simulink model "O_CloseLoop_Dynmodel"  (R2016b)
settings: Solver=VariableStepAuto  StartTime=0.0  StopTime=60.0  RelTol=1e-3
values from neighbouring files (symbols this model uses):
  MWS = JT9D_setup_everything_Dyn()    [BP_change_deter_data.m]    (also in JT9D_setup_everything_Dyn.m = input_set_0_0_100(MWS); make_train_data.m; sim_all_loss.m)
undefined symbols (not defined in the file or in its folder): Compressor, Lib_Turbo_Compressor_TMATS, stripchar_TMATS
libraries: Lib_Turbo_Duct_TMATS x5, Lib_Solve_DataOut_TMATS x5, Lib_Solve_OuterLoopIntegrator_TMATS x2, Lib_Turbo_Nozzle_TMATS x2, Lib_Turbo_Shaft_TMATS x2, Lib_Cntrl_FirstOrderActuator_TMATS x1, simulink x1, Lib_Cntrl_SimplePIcontroller_TMATS x1, Lib_Solve_IterNRSolverJC_TMATS x1, Lib_Turbo_Ambient_TMATS x1, Lib_Turbo_Burner_TMATS x1, Lib_Turbo_StaticCalc_TMATS x1
(part 2 of 2)

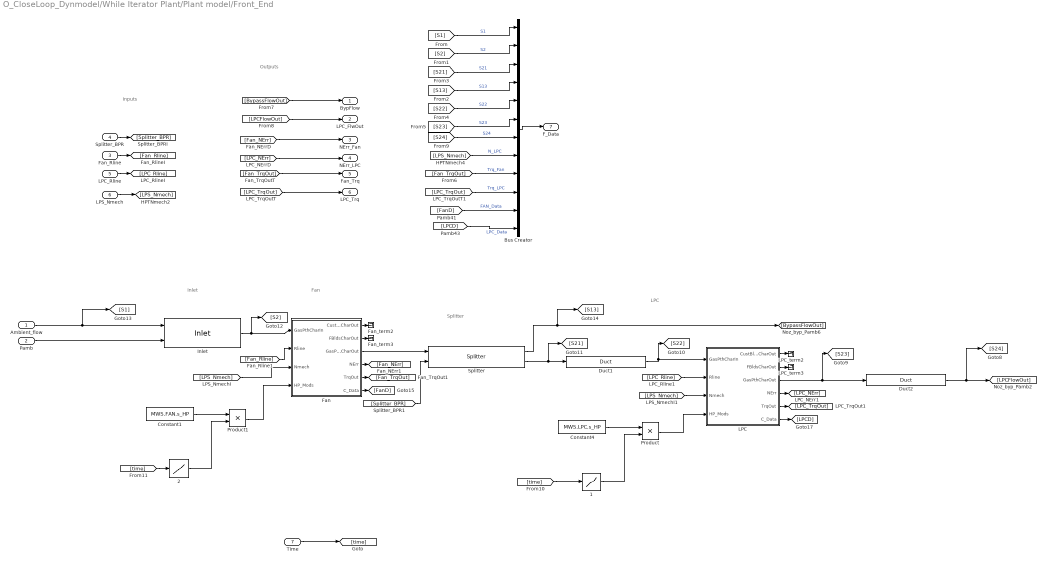
== system O_CloseLoop_Dynmodel/While Iterator Plant/Plant model/Front_End ==
  note: Inlet
  note: Fan
  note: Splitter
  note: LPC
  note: Outputs
  note: Inputs
  Ambient_flow : Inport
  Pamb : Inport  Port=2
  Fan_Rline : Inport  Port=3
  Splitter_BPR : Inport  Port=4
  LPC_Rline : Inport  Port=5
  LPS_Nmech : Inport  Port=6
  Time : Inport  Port=7
  1 : Lookup  InputValues=MWS.HP_in.t  Table=MWS.HP_in.scaled
  2 : Lookup  InputValues=MWS.HP_in.t  Table=MWS.HP_in.scaled
  Bus Creator : BusCreator  Inputs=12
  Constant1 : Constant  Value=MWS.FAN.s_HP
  Constant4 : Constant  Value=MWS.LPC.s_HP
  Duct1 : Lib_Turbo_Duct_TMATS/Duct  dP_M=MWS.Duct.dP1
  Duct2 : Lib_Turbo_Duct_TMATS/Duct  dP_M=MWS.Duct.dP2
  Fan : Subsystem  AncestorBlock=Lib_Turbo_Compressor_TMATS/Compressor  mask(T-MATS: Compressor Library Block){X_C_RlineVec_M=MWS.FAN.RlineVec, Z_C_AlphaVec_M=1, Y_C_Map_NcVec_M=MWS.FAN.NcVec, T_C_Map_WcArray_M=MWS.FAN.WcArray, T_C_Map_PRArray_M=MWS.FAN.PRArray, T_C_Map_EffArray_M=MWS.FAN.EffArray, s_C_Nc_M=MWS.FAN.s_Nc, s_C_Wc_M=MWS.FAN.s_Wc, s_C_PR_M=MWS.FAN.s_PR, s_C_Eff_M=MWS.FAN.s_eff, SL_M=off, Scale_M=none, CBLDEN_M=off, C_CBD_M=0, C_CBFht_M=0.5, C_CBFPt_M=0.5, FBLDEN_M=off, C_FBD_M=0, C_BFht_M=0.5, C_BFPt_M=0.5, DefSMEn_M=on, SRline_M=1, X_C_Map_WcSurgeVec_M=[0 200], T_C_Map_PRSurgeVec_M=[30 30], iDesign_M=MWS.iDes, NcDes_M=1, EffDes_M=0.8675, PRDes_M=1.645, RlineDes_M=2.3706, FVar_M=strcat('iDes_',stripchar_TMATS(gcb),'.bin'), BlkNm_M=double(gcb), HP_M=on}
      mask prompts: X_C_RlineVec_M "X_C_RlineVec_M - Compressor Map Rline Vector (X-axis)(nx1)"; Z_C_AlphaVec_M "Z_C_Map_AlphaVec_M - Compressor Alpha Vector (Z-axis)(rx1)"; Y_C_Map_NcVec_M "Y_C_Map_NcVec_M - Compressor Map Corrected Speed Vector (Y-axis)(mx1)"; T_C_Map_WcArray_M "T_C_Map_WcArray_M - Compressor Map Flow Array (Wc = f(Nc, Rline))(mxn)"; T_C_Map_PRArray_M "T_C_Map_PRArray_M - Compressor Map Pressure Ratio Array (PR = f(Nc, Rline))(mxn)"; T_C_Map_EffArray_M "T_C_Map_EffArray_M - Compressor Map Efficiency Array (Eff = f(Nc, Rline)(mxn)"; s_C_Nc_M "s_C_Nc_M - Corrected Speed Scalar Constant (C_Nc)"; s_C_Wc_M "s_C_Wc_M - Flow Scalar Constant (C_Wc)"; s_C_PR_M "s_C_PR_M - Pressure Ratio Scalar Constant (C_PR)"; s_C_Eff_M "s_C_Eff_M - Efficiency Scalar Constant (C_Eff)"; SL_M "Include surge line"; Scale_M "Scalars"; CBLDEN_M "CBLDEN_M - Customer Bleed Enable [0 - off, 1 - on]"; C_CBD_M "C_CBD_M - Customer or Flow based Bleed Demand[pps] (cbx1)"; C_CBFht_M "C_CBFht_M - Customer or Flow based Bleed Fractional enthalpy[frac] (cbx1)"; C_CBFPt_M "C_CBFPt_M - Customer or Flow based Bleed Fractional Total Pressure[frac] (cbx1)"; FBLDEN_M "FBLDEN_M - Fractional Bleed Enable [0 - off, 1 - on]"; C_FBD_M "C_FBD_M - Fractional Bleed Demand[frac] (bx1)"; C_BFht_M "C_BFht_M - Engine Bleed Fractional Enthalpy[frac] (bx1)"; C_BFPt_M "C_BFPt_M - Engine Bleed Fractional Total Pressure[frac] (bx1)"; DefSMEn_M "DefSMEn_M - Use map default (Rline = 1) surge line"; SRline_M "SRline_M - Rline defined as surge line"; X_C_Map_WcSurgeVec_M "X_C_Map_WcSurgeVec_M - map Compensated flow surge vector (sx1)"; T_C_Map_PRSurgeVec_M "T_C_Map_PRSurgeVec_M - map Surge Line Pressure Ratio vector (sx1)"; iDesign_M "iDesign_M - Design fork (0 - Enable iDes, 1 - Use iDes Scalars, 2 - Use Specified Input Scalars)"; NcDes_M "NcDes_M - map Design Corrected Shaft Speed [rpm]"; EffDes_M "EffDes_M  - Design Efficiency [frac]"; PRDes_M "PRDes_M - Design Pressure Ratio [frac]"; RlineDes_M "RlineDes_M - map Design Rline"; FVar_M "FVar_M - File name for iDes Variables"; BlkNm_M "Block name as double for Simulink output"; HP_M "HP_M - Enable Health Parameter input (3x1 vector)"
      mask help: This block simulates the performance of a compressor using basic thermodynamic equations, properties, and table lookups.
      mask init:
      | MSK_CompInit_TMATS
      mask Help: web(which('Turbo_TMATS_Cmp.html'),'-helpbrowser')
      mask TypeOptions Scale_M: none | user defined | iDesign
      mask Callback CBLDEN_M: MSK_SEC_Enables_TMATS('CBLDEN_M',[14 15 16],'en')
      mask Callback FBLDEN_M: MSK_SEC_Enables_TMATS('FBLDEN_M',[18 19 20],'en')
      mask Callback DefSMEn_M:
      | MSK_SEC_Enables_TMATS('DefSMEn_M',[23 24],'dis')
      | MSK_SEC_Enables_TMATS('DefSMEn_M',[22],'en')
      mask Callback iDesign_M:
      | MSK_SEC_Enables_Ides_TMATS('iDesign_M',[7 8 9 10],'G1')
      | MSK_SEC_Enables_Ides_TMATS('iDesign_M',[26 27 28 29],'G2')
      | MSK_SEC_Enables_Ides_TMATS('iDesign_M',[30],'G3')
      mask DialogControl Control2 Prompt: Plot Map
      mask DialogControl Control2 Callback: MSK_PlotCMap_TMATS()
  Fan_term2 : Terminator
  Fan_term3 : Terminator
  Inlet : Lib_Turbo_Inlet_TMATS/Inlet  eRambase_M=MWS.Inlet.eRamBase  X_eRamVec_M=MWS.Inlet.eRamVec  T_eRamtbl_M=MWS.Inlet.eRamtbl
  LPC : Subsystem  mask(T-MATS: Compressor Library Block){X_C_RlineVec_M=MWS.LPC.RlineVec, Z_C_AlphaVec_M=1, Y_C_Map_NcVec_M=MWS.LPC.NcVec, T_C_Map_WcArray_M=MWS.LPC.WcArray, T_C_Map_PRArray_M=MWS.LPC.PRArray, T_C_Map_EffArray_M=MWS.LPC.EffArray, s_C_Nc_M=MWS.LPC.s_Nc, s_C_Wc_M=MWS.LPC.s_Wc, s_C_PR_M=MWS.LPC.s_PR, s_C_Eff_M=MWS.LPC.s_eff, SL_M=off, Scale_M=none, CBLDEN_M=off, C_CBD_M=0, C_CBFht_M=0.5, C_CBFPt_M=0.5, FBLDEN_M=off, C_FBD_M=0, C_BFht_M=0.5, C_BFPt_M=0.5, DefSMEn_M=on, SRline_M=1, X_C_Map_WcSurgeVec_M=[0 200], T_C_Map_PRSurgeVec_M=[30 30], iDesign_M=MWS.iDes, NcDes_M=0.993, EffDes_M=.8683, PRDes_M=2.488, RlineDes_M=1.7664, FVar_M=strcat('iDes_',stripchar_TMATS(gcb),'.bin'), BlkNm_M=double(gcb), HP_M=on}
      mask prompts: X_C_RlineVec_M "X_C_RlineVec_M - Compressor Map Rline Vector (X-axis)(nx1)"; Z_C_AlphaVec_M "Z_C_Map_AlphaVec_M - Compressor Alpha Vector (Z-axis)(rx1)"; Y_C_Map_NcVec_M "Y_C_Map_NcVec_M - Compressor Map Corrected Speed Vector (Y-axis)(mx1)"; T_C_Map_WcArray_M "T_C_Map_WcArray_M - Compressor Map Flow Array (Wc = f(Nc, Rline))(mxn)"; T_C_Map_PRArray_M "T_C_Map_PRArray_M - Compressor Map Pressure Ratio Array (PR = f(Nc, Rline))(mxn)"; T_C_Map_EffArray_M "T_C_Map_EffArray_M - Compressor Map Efficiency Array (Eff = f(Nc, Rline)(mxn)"; s_C_Nc_M "s_C_Nc_M - Corrected Speed Scalar Constant (C_Nc)"; s_C_Wc_M "s_C_Wc_M - Flow Scalar Constant (C_Wc)"; s_C_PR_M "s_C_PR_M - Pressure Ratio Scalar Constant (C_PR)"; s_C_Eff_M "s_C_Eff_M - Efficiency Scalar Constant (C_Eff)"; SL_M "Include surge line"; Scale_M "Scalars"; CBLDEN_M "CBLDEN_M - Customer Bleed Enable [0 - off, 1 - on]"; C_CBD_M "C_CBD_M - Customer or Flow based Bleed Demand[pps] (cbx1)"; C_CBFht_M "C_CBFht_M - Customer or Flow based Bleed Fractional enthalpy[frac] (cbx1)"; C_CBFPt_M "C_CBFPt_M - Customer or Flow based Bleed Fractional Total Pressure[frac] (cbx1)"; FBLDEN_M "FBLDEN_M - Fractional Bleed Enable [0 - off, 1 - on]"; C_FBD_M "C_FBD_M - Fractional Bleed Demand[frac] (bx1)"; C_BFht_M "C_BFht_M - Engine Bleed Fractional Enthalpy[frac] (bx1)"; C_BFPt_M "C_BFPt_M - Engine Bleed Fractional Total Pressure[frac] (bx1)"; DefSMEn_M "DefSMEn_M - Use map default (Rline = 1) surge line"; SRline_M "SRline_M - Rline defined as surge line"; X_C_Map_WcSurgeVec_M "X_C_Map_WcSurgeVec_M - map Compensated flow surge vector (sx1)"; T_C_Map_PRSurgeVec_M "T_C_Map_PRSurgeVec_M - map Surge Line Pressure Ratio vector (sx1)"; iDesign_M "iDesign_M - Design fork (0 - Enable iDes, 1 - Use iDes Scalars, 2 - Use Specified Input Scalars)"; NcDes_M "NcDes_M - map Design Corrected Shaft Speed [rpm]"; EffDes_M "EffDes_M  - Design Efficiency [frac]"; PRDes_M "PRDes_M - Design Pressure Ratio [frac]"; RlineDes_M "RlineDes_M - map Design Rline"; FVar_M "FVar_M - File name for iDes Variables"; BlkNm_M "Block name as double for Simulink output"; HP_M "HP_M - Enable Health Parameter input (3x1 vector)"
      mask help: This block simulates the performance of a compressor using basic thermodynamic equations, properties, and table lookups.
      mask init:
      | MSK_CompInit_TMATS
      mask Help: web(which('Turbo_TMATS_Cmp.html'),'-helpbrowser')
      mask TypeOptions Scale_M: none | user defined | iDesign
      mask Callback CBLDEN_M: MSK_SEC_Enables_TMATS('CBLDEN_M',[14 15 16],'en')
      mask Callback FBLDEN_M: MSK_SEC_Enables_TMATS('FBLDEN_M',[18 19 20],'en')
      mask Callback DefSMEn_M:
      | MSK_SEC_Enables_TMATS('DefSMEn_M',[23 24],'dis')
      | MSK_SEC_Enables_TMATS('DefSMEn_M',[22],'en')
      mask Callback iDesign_M:
      | MSK_SEC_Enables_Ides_TMATS('iDesign_M',[7 8 9 10],'G1')
      | MSK_SEC_Enables_Ides_TMATS('iDesign_M',[26 27 28 29],'G2')
      | MSK_SEC_Enables_Ides_TMATS('iDesign_M',[30],'G3')
      mask DialogControl Control2 Prompt: Plot Map
      mask DialogControl Control2 Callback: MSK_PlotCMap_TMATS()
  LPC_term2 : Terminator
  LPC_term3 : Terminator
  Product : Product
  Product1 : Product
  Splitter : Lib_Turbo_Splitter_TMATS/Splitter
  BypFlow : Outport
  LPC_FlwOut : Outport  Port=2
  NErr_Fan : Outport  Port=3
  NErr_LPC : Outport  Port=4
  Fan_Trq : Outport  Port=5
  LPC_Trq : Outport  Port=6
  F_Data : Outport  Port=7
  wires:
  [LPCFlowOut] -> LPC_FlwOut/1
  [Splitter_BPR] -> Splitter/2
  Inlet/1 -> [S2], Fan/1(GasPthCharIn)
  [Fan_Rline] -> Fan/2(Rline)
  LPC/2(FBldsCharOut) -> LPC_term3/1
  LPC/4(NErr) -> [LPC_NErr]
  LPC/5(TrqOut) -> [LPC_TrqOut]
  LPC/1(CustBldsCharOut) -> LPC_term2/1
  [LPC_Rline] -> LPC/2(Rline)
  Fan/2(FBldsCharOut) -> Fan_term3/1
  Fan/6(C_Data) -> [FanD]
  Fan/1(CustBldsCharOut) -> Fan_term2/1
  Fan/5(TrqOut) -> [Fan_TrqOut]
  Fan/4(NErr) -> [Fan_NErr]
  Duct1/1 -> LPC/1(GasPthCharIn), [S22]
  Splitter/2 -> [S21], Duct1/1
  Fan/3(GasPthCharOut) -> Splitter/1
  [LPS_Nmech] -> LPC/3(Nmech)
  [LPS_Nmech] -> Fan/3(Nmech)
  [Fan_TrqOut] -> Bus Creator/9  "Trq_Fan"
  LPC/6(C_Data) -> [LPCD]
  Pamb/1 -> Inlet/2
  Ambient_flow/1 -> [S1], Inlet/1
  Fan_Rline/1 -> [Fan_Rline]
  LPS_Nmech/1 -> [LPS_Nmech]
  Splitter_BPR/1 -> [Splitter_BPR]
  LPC_Rline/1 -> [LPC_Rline]
  [S1] -> Bus Creator/1  "S1"
  [FanD] -> Bus Creator/11  "FAN_Data"
  [S22] -> Bus Creator/5  "S22"
  [S23] -> Bus Creator/6  "S23"
  [S21] -> Bus Creator/3  "S21"
  Bus Creator/1 -> F_Data/1
  [LPC_TrqOut] -> Bus Creator/10  "Trq_LPC"
  [LPCD] -> Bus Creator/12  "LPC_Data"
  [S2] -> Bus Creator/2  "S2"
  [LPS_Nmech] -> Bus Creator/8  "N_LPC"
  [S13] -> Bus Creator/4  "S13"
  Splitter/1 -> [S13], [BypassFlowOut]
  LPC/3(GasPthCharOut) -> Duct2/1, [S23]
  [LPC_TrqOut] -> LPC_Trq/1
  [Fan_NErr] -> NErr_Fan/1
  [Fan_TrqOut] -> Fan_Trq/1
  [LPC_NErr] -> NErr_LPC/1
  [BypassFlowOut] -> BypFlow/1
  Duct2/1 -> [LPCFlowOut], [S24]
  [S24] -> Bus Creator/7  "S24"
  Constant4/1 -> Product/1
  Product/1 -> LPC/4(HP_Mods)
  1/1 -> Product/2
  [time] -> 1/1
  Time/1 -> [time]
  Constant1/1 -> Product1/1
  Product1/1 -> Fan/4(HP_Mods)
  2/1 -> Product1/2
  [time] -> 2/1

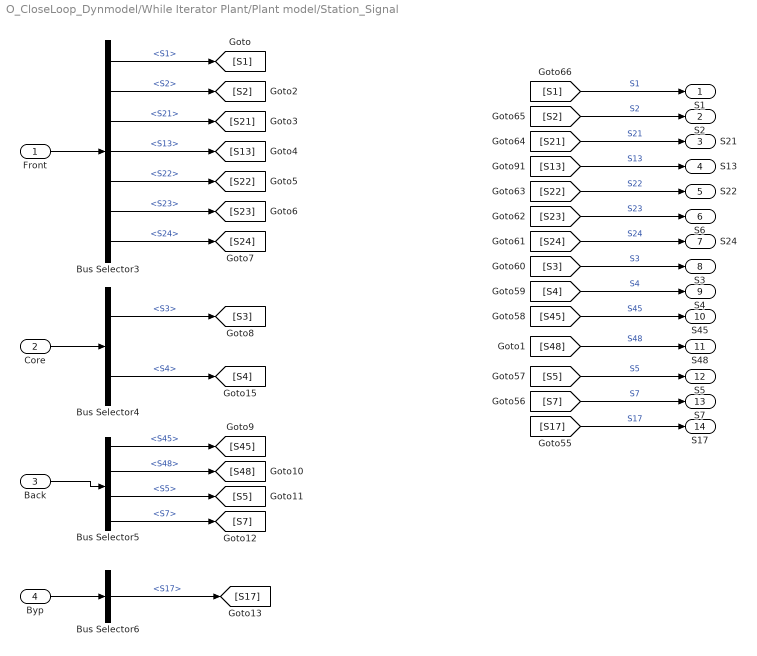
== system O_CloseLoop_Dynmodel/While Iterator Plant/Plant model/Station_Signal ==
  Front : Inport
  Core : Inport  Port=2
  Back : Inport  Port=3
  Byp : Inport  Port=4
  Bus Selector3 : BusSelector  OutputSignals=S1,S2,S21,S13,S22,S23,S24
  Bus Selector4 : BusSelector  OutputSignals=S3,S4
  Bus Selector5 : BusSelector  OutputSignals=S45,S48,S5,S7
  Bus Selector6 : BusSelector  OutputSignals=S17
  S1 : Outport
  S2 : Outport  Port=2
  S21 : Outport  Port=3
  S13 : Outport  Port=4
  S22 : Outport  Port=5
  S6 : Outport  Port=6
  S24 : Outport  Port=7
  S3 : Outport  Port=8
  S4 : Outport  Port=9
  S45 : Outport  Port=10
  S48 : Outport  Port=11
  S5 : Outport  Port=12
  S7 : Outport  Port=13
  S17 : Outport  Port=14
  wires:
  [S21] -> S21/1  "S21"
  [S45] -> S45/1  "S45"
  [S23] -> S6/1  "S23"
  [S7] -> S7/1  "S7"
  [S13] -> S13/1  "S13"
  [S22] -> S22/1  "S22"
  [S3] -> S3/1  "S3"
  [S4] -> S4/1  "S4"
  [S5] -> S5/1  "S5"
  [S17] -> S17/1  "S17"
  [S2] -> S2/1  "S2"
  [S24] -> S24/1  "S24"
  [S1] -> S1/1  "S1"
  Bus Selector4/2 -> [S4]  "<S4>"
  Bus Selector5/4 -> [S7]  "<S7>"
  Core/1 -> Bus Selector4/1
  Bus Selector5/1 -> [S45]  "<S45>"
  Bus Selector6/1 -> [S17]  "<S17>"
  Byp/1 -> Bus Selector6/1
  Bus Selector4/1 -> [S3]  "<S3>"
  Back/1 -> Bus Selector5/1
  Bus Selector5/2 -> [S48]  "<S48>"
  Bus Selector5/3 -> [S5]  "<S5>"
  [S48] -> S48/1  "S48"
  Bus Selector3/4 -> [S13]  "<S13>"
  Bus Selector3/5 -> [S22]  "<S22>"
  Bus Selector3/7 -> [S24]  "<S24>"
  Bus Selector3/3 -> [S21]  "<S21>"
  Bus Selector3/2 -> [S2]  "<S2>"
  Bus Selector3/6 -> [S23]  "<S23>"
  Front/1 -> Bus Selector3/1
  Bus Selector3/1 -> [S1]  "<S1>"

== system O_CloseLoop_Dynmodel/While Iterator Plant/Plant model/Subsystem ==
  BypFlow : Inport
  Pamb : Inport  Port=2
  Bus Creator8 : BusCreator  Inputs=2
  Duct5 : Lib_Turbo_Duct_TMATS/Duct  dP_M=MWS.Duct.dP5
  Noz_byp : Lib_Turbo_Nozzle_TMATS/Nozzle  SWType_M=Convergent  N_TArea_M=MWS.NozB.Ath  N_EArea_M=110.7  N_FL_M=0.00  X_N_TtVec2_M=[300 2000]  T_N_TGArray_M=[1 1]  X_N_PEQPaVec_M=[0 10000]  T_N_CdThArray_M=[1 1]  T_N_CvArray_M=MWS.NozB.CvArray  CfgEn_M=off  T_N_CfgArray_M=[1 1]  X_N_FARVec_M=[0; 0.0050; 0.0100; 0.0150; 0.0200; 0.0250; 0.0300]  T_N_RtArray_M="[0.0686;    0.0686;    0.0686;    0.0686;    0.0686;    0.0686;    0.0686]"  Y_N_TtVec_M=[300 2000]  T_N_MAP_gammaArray_M=[ 1.4 1.4 1.4 1.4 1.4 1.4 1.4; 1.4 1.4 1.4 1.4 1.4 1.4 1.4]  iDesign_M=MWS.iDes  WDes_M=562.61  FVar_M=strcat('iDes_',stripchar_TMATS(gcb),'.bin')
  Noz_byp_term1 : Terminator
  Noz_byp_term3 : Terminator
  NErr_Noz_byp : Outport
  By_Data : Outport  Port=2
  wires:
  Pamb/1 -> Noz_byp/2
  Duct5/1 -> [S17], Noz_byp/1
  Noz_byp/4 -> Noz_byp_term1/1
  Noz_byp/3 -> [Noz_byp_NErr]
  Noz_byp/1 -> Noz_byp_term3/1
  Noz_byp/2 -> [Byp_Fg]
  BypFlow/1 -> Duct5/1
  [S17] -> Bus Creator8/1  "S17"
  Bus Creator8/1 -> By_Data/1
  [Noz_byp_NErr] -> NErr_Noz_byp/1
  [Byp_Fg] -> Bus Creator8/2  "Fg_Byp"

== system O_CloseLoop_Dynmodel/While Iterator Plant/Plant model/Thrust_Calculate ==
  Byp_Fg : Inport
  Core_Fg : Inport  Port=2
  AmbData : Inport  Port=3
  Wf : Inport  Port=4
  Bus Selector : BusSelector  OutputSignals=Fdrag
  Compressor_term1 : Terminator
  Display1 : Display
  Display2 : Display
  Display3 : Display
  SFCCalc : Lib_Turbo_SFCCalc_TMATS/SFCCalc
  Scope1 : Scope
  Scope2 : Scope
  Sum : Sum  Inputs=|++
  Fg : Outport
  TSFC : Outport  Port=2
  Fnet : Outport  Port=3
  wires:
  [Fg] -> Fg/1
  [TSFC] -> TSFC/1
  Core_Fg/1 -> [Core_Fg]
  AmbData/1 -> [AmbData]
  SFCCalc/1 -> [TSFC]
  [Wf] -> SFCCalc/1
  [TSFC] -> Display3/1, Compressor_term1/1
  [Byp_Fg] -> Sum/1
  Sum/1 -> Display2/1, [Fg]
  [AmbData] -> Bus Selector/1
  Bus Selector/1 -> Scope2/1, SFCCalc/3  "<Fdrag>"
  SFCCalc/2 -> Display1/1, Scope1/1, [Fnet]
  [Core_Fg] -> Sum/2
  [Fg] -> SFCCalc/2
  Byp_Fg/1 -> [Byp_Fg]
  Wf/1 -> [Wf]
  [Fnet] -> Fnet/1

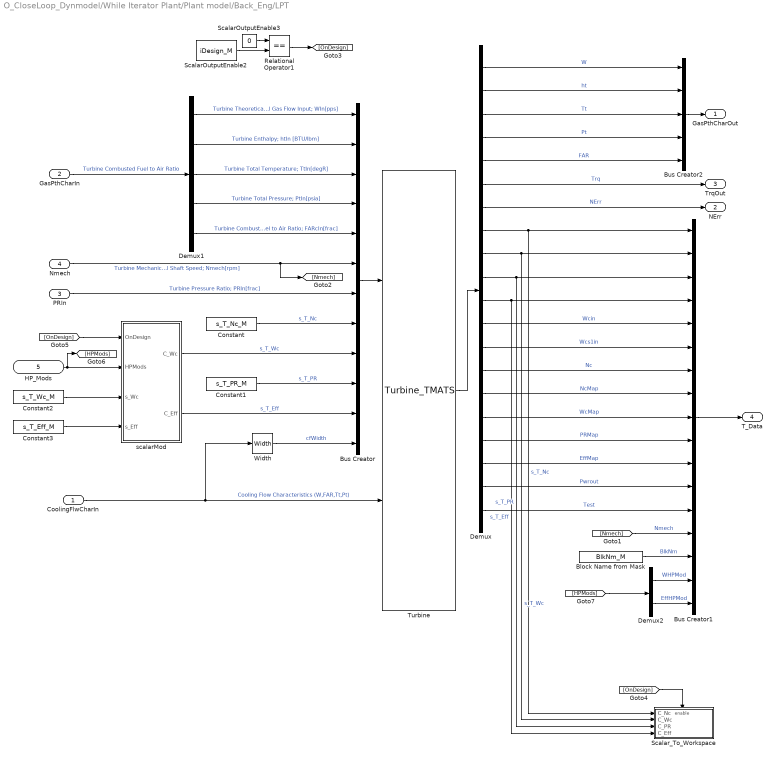
== system O_CloseLoop_Dynmodel/While Iterator Plant/Plant model/Back_Eng/LPT ==
  CoolingFlwCharIn : Inport
  GasPthCharIn : Inport  Port=2
  PRIn : Inport  Port=3
  Nmech : Inport  Port=4
  HP_Mods : Inport  Port=5
  Block Name from Mask : Constant  Value=BlkNm_M
  Bus Creator : BusCreator  Inputs=12
  Bus Creator1 : BusCreator  Inputs=17
  Bus Creator2 : BusCreator  Inputs=5
  Constant : Constant  Value=s_T_Nc_M
  Constant1 : Constant  Value=s_T_PR_M
  Constant2 : Constant  Value=s_T_Wc_M
  Constant3 : Constant  Value=s_T_Eff_M
  Demux : Demux  Outputs=20
  Demux1 : Demux  Outputs=5
  Demux2 : Demux  Outputs=2
  Relational Operator1 : RelationalOperator  Operator===  OutDataTypeStr=boolean  RndMeth=Nearest
  ScalarOutputEnable2 : Constant  Value=iDesign_M
  ScalarOutputEnable3 : Constant  Value=0
  Scalar_To_Workspace : Subsystem
  Turbine : S-Function  FunctionName=Turbine_TMATS  Parameters=Y_T_Map_NcVec_M, X_T_Map_PRVec_M, T_T_Map_WcArray_M, T_T_Map_EffArray_M, T_CoolFlwPos_M, length(T_CoolFlwPos_M), CFlwEn_M, iDesign_M, NcDes_M, EffDes_M, PRDes_M, NDes_M, gcs, size(T_T_Map_WcArray_M,2), size(T_T_Map_EffArray_M,2), size(T_T_Map_WcArray_M,1), size(T_T_Map_EffArray_M,1), ConfigNPSS_M  SFunctionModules='h2tc_TMATS pt2sc_TMATS sp2tc_TMATS t2hc_TMATS interp2Ac_TMATS functions_TMATS'  SFunctionDeploymentMode=off  EnableBusSupport=off
  Width : Width
  scalarMod : Subsystem
  GasPthCharOut : Outport
  NErr : Outport  Port=2
  TrqOut : Outport  Port=3
  T_Data : Outport  Port=4
  wires:
  [HPMods] -> Demux2/1
  Demux2/2 -> Bus Creator1/17  "EffHPMod"
  Demux2/1 -> Bus Creator1/16  "WHPMod"
  Constant3/1 -> scalarMod/4(s_Eff)
  Constant2/1 -> scalarMod/3(s_Wc)
  [OnDesign] -> scalarMod/1(OnDesign)
  HP_Mods/1 -> scalarMod/2(HPMods), [HPMods]
  [OnDesign] -> Scalar_To_Workspace/Enable
  Relational Operator1/1 -> [OnDesign]
  ScalarOutputEnable3/1 -> Relational Operator1/1
  ScalarOutputEnable2/1 -> Relational Operator1/2
  scalarMod/2(C_Eff) -> Bus Creator/11  "s_T_Eff"
  scalarMod/1(C_Wc) -> Bus Creator/9  "s_T_Wc"
  Constant1/1 -> Bus Creator/10  "s_T_PR"
  Constant/1 -> Bus Creator/8  "s_T_Nc"
  [Nmech] -> Bus Creator1/14  "Nmech"
  Block Name from Mask/1 -> Bus Creator1/15  "BlkNm"
  Demux/12 -> Bus Creator1/5  "Wcin"
  PRIn/1 -> Bus Creator/7  "Turbine Pressure Ratio; PRIn[frac]"
  Demux1/2 -> Bus Creator/2  "Turbine Enthalpy; htIn [BTU/lbm]"
  Demux1/3 -> Bus Creator/3  "Turbine Total Temperature; TtIn[degR]"
  Turbine/1 -> Demux/1
  Demux/1 -> Bus Creator2/1  "W"
  Demux/5 -> Bus Creator2/5  "FAR"
  Demux/3 -> Bus Creator2/3  "Tt"
  Demux/4 -> Bus Creator2/4  "Pt"
  Bus Creator/1 -> Turbine/1
  Demux/2 -> Bus Creator2/2  "ht"
  Demux/6 -> TrqOut/1  "Trq"
  Nmech/1 -> Bus Creator/6, [Nmech]  "Turbine Mechanical Shaft Speed; Nmech[rpm]"
  Demux1/4 -> Bus Creator/4  "Turbine Total Pressure; PtIn[psia]"
  Bus Creator2/1 -> GasPthCharOut/1
  GasPthCharIn/1 -> Demux1/1  "Turbine Combusted Fuel to Air Ratio"
  Demux1/1 -> Bus Creator/1  "Turbine Theoretical Gas Flow Input; WIn[pps]"
  Demux/7 -> NErr/1  "NErr"
  CoolingFlwCharIn/1 -> Width/1, Turbine/2  "Cooling Flow Characteristics (W,FAR,Tt,Pt)"
  Demux1/5 -> Bus Creator/5  "Turbine Combusted Fuel to Air Ratio; FARcIn[frac]"
  Bus Creator1/1 -> T_Data/1
  Demux/8 -> Scalar_To_Workspace/1(C_Nc), Bus Creator1/1  "s_T_Nc"
  Demux/9 -> Scalar_To_Workspace/2(C_Wc), Bus Creator1/2  "s_T_Wc"
  Demux/10 -> Scalar_To_Workspace/3(C_PR), Bus Creator1/3  "s_T_PR"
  Demux/11 -> Scalar_To_Workspace/4(C_Eff), Bus Creator1/4  "s_T_Eff"
  Width/1 -> Bus Creator/12  "cfWidth"
  Demux/20 -> Bus Creator1/13  "Test"
  Demux/13 -> Bus Creator1/6  "Wcs1in"
  Demux/14 -> Bus Creator1/7  "Nc"
  Demux/15 -> Bus Creator1/8  "NcMap"
  Demux/16 -> Bus Creator1/9  "WcMap"
  Demux/17 -> Bus Creator1/10  "PRMap"
  Demux/18 -> Bus Creator1/11  "EffMap"
  Demux/19 -> Bus Creator1/12  "Pwrout"

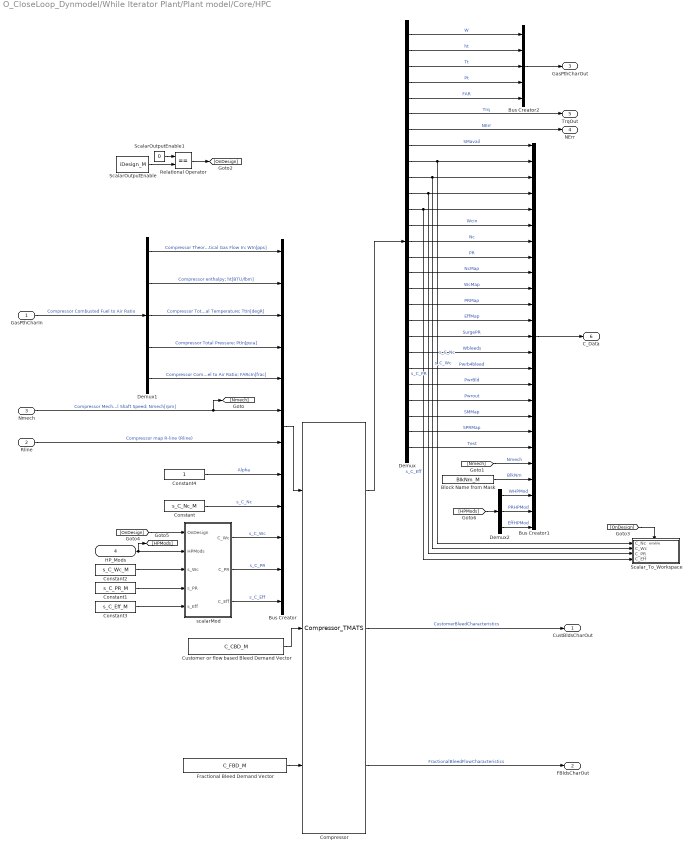
== system O_CloseLoop_Dynmodel/While Iterator Plant/Plant model/Core/HPC ==
  GasPthCharIn : Inport
  Rline : Inport  Port=2
  Nmech : Inport  Port=3
  HP_Mods : Inport  Port=4
  Block Name from Mask : Constant  Value=BlkNm_M
  Bus Creator : BusCreator  Inputs=12
  Bus Creator1 : BusCreator  Inputs=25
  Bus Creator2 : BusCreator  Inputs=5
  Compressor : S-Function  FunctionName=Compressor_TMATS  Parameters="Y_C_Map_NcVec_M, X_C_RlineVec_M, Z_C_AlphaVec_M, T_C_Map_WcArray_M, T_C_Map_PRArray_M, T_C_Map_EffArray_M, C_CBFht_M, C_CBFPt_M,  C_BFht_M, C_BFPt_M, X_C_Map_WcSurgeVec_M, T_C_Map_PRSurgeVec_M, iDesign_M, NcDes_M, EffDes_M, PRDes_M, RlineDes_M, CBLDEN_M, FBLDEN_M, gcs, length(C_CBD_M), length(C_FBD_M), size(T_C_Map_WcArray_M,2), size(T_C_Map_PRArray_M,2), size(T_C_Map_EffArray_M,2), size(T_C_Map_WcArray_M,1), size(T_C_Map_PRArray_M,1), size(T_C_Map_EffArray_M,1), size(T_C_Map_WcArray_M,3), size(T_C_Map_PRArray_M,3), size(T_C_Map_EffArray_M,3)"  SFunctionModules='h2tc_TMATS pt2sc_TMATS sp2tc_TMATS t2hc_TMATS interp1Ac_TMATS interp2Ac_TMATS interp3Ac_TMATS functions_TMATS'  SFunctionDeploymentMode=off  EnableBusSupport=off
  Constant : Constant  Value=s_C_Nc_M
  Constant1 : Constant  Value=s_C_PR_M
  Constant2 : Constant  Value=s_C_Wc_M
  Constant3 : Constant  Value=s_C_Eff_M
  Constant4 : Constant
  Customer or flow based Bleed Demand Vector : Constant  Value=C_CBD_M
  Demux : Demux  Outputs=27
  Demux1 : Demux  Outputs=5
  Demux2 : Demux  Outputs=3
  Fractional Bleed Demand Vector : Constant  Value=C_FBD_M
  Relational Operator : RelationalOperator  Operator===  OutDataTypeStr=boolean  RndMeth=Nearest
  ScalarOutputEnable : Constant  Value=iDesign_M
  ScalarOutputEnable1 : Constant  Value=0
  Scalar_To_Workspace : Subsystem
  scalarMod : Subsystem
  CustBldsCharOut : Outport  PortDimensions=length(C_CBD_M)*5
  FBldsCharOut : Outport  Port=2  PortDimensions=length(C_FBD_M)*5
  GasPthCharOut : Outport  Port=3
  NErr : Outport  Port=4
  TrqOut : Outport  Port=5
  C_Data : Outport  Port=6
  wires:
  [HPMods] -> Demux2/1
  Demux2/1 -> Bus Creator1/23  "WHPMod"
  Demux2/3 -> Bus Creator1/25  "EffHPMod"
  Demux2/2 -> Bus Creator1/24  "PRHPMod"
  [OnDesign] -> scalarMod/1(OnDesign)
  HP_Mods/1 -> scalarMod/2(HPMods), [HPMods]
  scalarMod/3(C_Eff) -> Bus Creator/12  "s_C_Eff"
  scalarMod/2(C_PR) -> Bus Creator/11  "s_C_PR"
  scalarMod/1(C_Wc) -> Bus Creator/10  "s_C_Wc"
  Constant3/1 -> scalarMod/5(s_Eff)
  Constant1/1 -> scalarMod/4(s_PR)
  Constant2/1 -> scalarMod/3(s_Wc)
  [OnDesign] -> Scalar_To_Workspace/Enable
  Constant4/1 -> Bus Creator/8  "Alpha"
  Constant/1 -> Bus Creator/9  "s_C_Nc"
  Block Name from Mask/1 -> Bus Creator1/22  "BlkNm"
  [Nmech] -> Bus Creator1/21  "Nmech"
  Demux/27 -> Bus Creator1/20  "Test"
  Demux/26 -> Bus Creator1/19  "SPRMap"
  Demux/25 -> Bus Creator1/18  "SMMap"
  Demux/18 -> Bus Creator1/11  "PRMap"
  Demux/15 -> Bus Creator1/8  "PR"
  Demux/17 -> Bus Creator1/10  "WcMap"
  Demux/19 -> Bus Creator1/12  "EffMap"
  Demux/24 -> Bus Creator1/17  "Pwrout"
  Demux/16 -> Bus Creator1/9  "NcMap"
  Demux/20 -> Bus Creator1/13  "SurgePR"
  Demux/21 -> Bus Creator1/14  "Wbleeds"
  Demux/22 -> Bus Creator1/15  "Pwrb4bleed"
  Demux/23 -> Bus Creator1/16  "PwrBld"
  Demux/14 -> Bus Creator1/7  "Nc"
  Relational Operator/1 -> [OnDesign]
  ScalarOutputEnable1/1 -> Relational Operator/1
  ScalarOutputEnable/1 -> Relational Operator/2
  Demux/12 -> Bus Creator1/5, Scalar_To_Workspace/4(C_Eff)  "s_C_Eff"
  Demux/11 -> Bus Creator1/4, Scalar_To_Workspace/3(C_PR)  "s_C_PR"
  Demux/10 -> Bus Creator1/3, Scalar_To_Workspace/2(C_Wc)  "s_C_Wc"
  Demux/9 -> Bus Creator1/2, Scalar_To_Workspace/1(C_Nc)  "s_C_Nc"
  Bus Creator1/1 -> C_Data/1
  Demux/8 -> Bus Creator1/1  "SMavail"
  Demux1/2 -> Bus Creator/2  "Compressor enthalpy; ht[BTU/lbm]"
  Compressor/3 -> FBldsCharOut/1  "FractionalBleedFlowCharacteristics"
  Compressor/2 -> CustBldsCharOut/1  "CustomerBleedCharacteristics"
  Fractional Bleed Demand Vector/1 -> Compressor/3
  Customer or flow based Bleed Demand Vector/1 -> Compressor/2
  Demux/7 -> NErr/1  "NErr"
  Demux1/1 -> Bus Creator/1  "Compressor Theoretical Gas Flow In; WIn[pps]"
  GasPthCharIn/1 -> Demux1/1  "Compressor Combusted Fuel to Air Ratio"
  Bus Creator2/1 -> GasPthCharOut/1
  Demux/2 -> Bus Creator2/2  "ht"
  Demux/13 -> Bus Creator1/6  "Wcin"
  Rline/1 -> Bus Creator/7  "Compressor map R-line (Rline)"
  Demux1/5 -> Bus Creator/5  "Compressor Combusted Fuel to Air Ratio; FARcIn[frac]"
  Demux1/3 -> Bus Creator/3  "Compressor Total Temperature; TtIn[degR]"
  Compressor/1 -> Demux/1
  Demux/1 -> Bus Creator2/1  "W"
  Demux/5 -> Bus Creator2/5  "FAR"
  Demux/3 -> Bus Creator2/3  "Tt"
  Demux/4 -> Bus Creator2/4  "Pt"
  Bus Creator/1 -> Compressor/1
  Demux/6 -> TrqOut/1  "Trq"
  Nmech/1 -> Bus Creator/6, [Nmech]  "Compressor Mechanical Shaft Speed; Nmech[rpm]"
  Demux1/4 -> Bus Creator/4  "Compressor Total Pressure; PtIn[psia]"

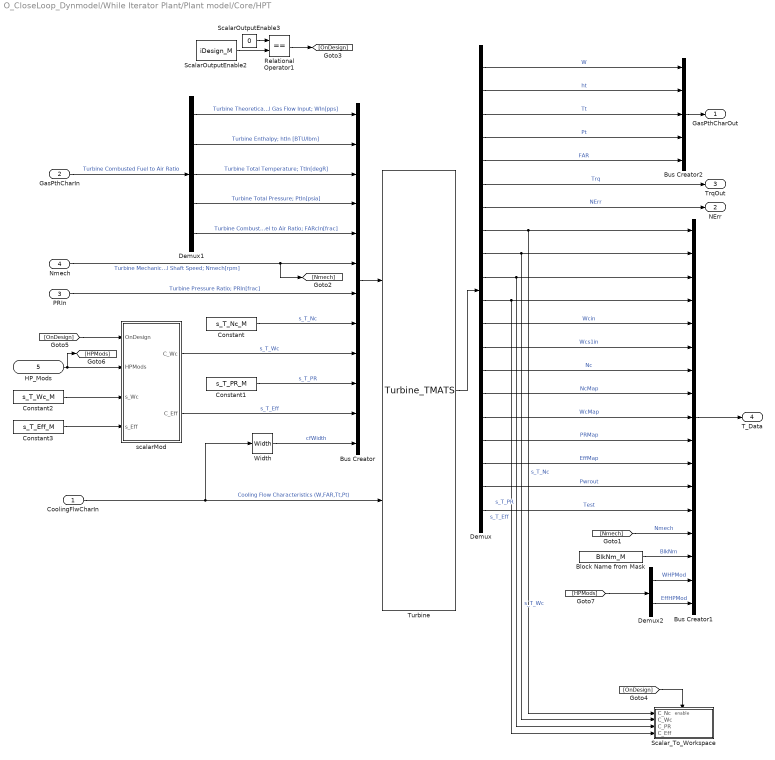
== system O_CloseLoop_Dynmodel/While Iterator Plant/Plant model/Core/HPT ==
  CoolingFlwCharIn : Inport
  GasPthCharIn : Inport  Port=2
  PRIn : Inport  Port=3
  Nmech : Inport  Port=4
  HP_Mods : Inport  Port=5
  Block Name from Mask : Constant  Value=BlkNm_M
  Bus Creator : BusCreator  Inputs=12
  Bus Creator1 : BusCreator  Inputs=17
  Bus Creator2 : BusCreator  Inputs=5
  Constant : Constant  Value=s_T_Nc_M
  Constant1 : Constant  Value=s_T_PR_M
  Constant2 : Constant  Value=s_T_Wc_M
  Constant3 : Constant  Value=s_T_Eff_M
  Demux : Demux  Outputs=20
  Demux1 : Demux  Outputs=5
  Demux2 : Demux  Outputs=2
  Relational Operator1 : RelationalOperator  Operator===  OutDataTypeStr=boolean  RndMeth=Nearest
  ScalarOutputEnable2 : Constant  Value=iDesign_M
  ScalarOutputEnable3 : Constant  Value=0
  Scalar_To_Workspace : Subsystem
  Turbine : S-Function  FunctionName=Turbine_TMATS  Parameters=Y_T_Map_NcVec_M, X_T_Map_PRVec_M, T_T_Map_WcArray_M, T_T_Map_EffArray_M, T_CoolFlwPos_M, length(T_CoolFlwPos_M), CFlwEn_M, iDesign_M, NcDes_M, EffDes_M, PRDes_M, NDes_M, gcs, size(T_T_Map_WcArray_M,2), size(T_T_Map_EffArray_M,2), size(T_T_Map_WcArray_M,1), size(T_T_Map_EffArray_M,1), ConfigNPSS_M  SFunctionModules='h2tc_TMATS pt2sc_TMATS sp2tc_TMATS t2hc_TMATS interp2Ac_TMATS functions_TMATS'  SFunctionDeploymentMode=off  EnableBusSupport=off
  Width : Width
  scalarMod : Subsystem
  GasPthCharOut : Outport
  NErr : Outport  Port=2
  TrqOut : Outport  Port=3
  T_Data : Outport  Port=4
  wires:
  [HPMods] -> Demux2/1
  Demux2/2 -> Bus Creator1/17  "EffHPMod"
  Demux2/1 -> Bus Creator1/16  "WHPMod"
  Constant3/1 -> scalarMod/4(s_Eff)
  Constant2/1 -> scalarMod/3(s_Wc)
  [OnDesign] -> scalarMod/1(OnDesign)
  HP_Mods/1 -> scalarMod/2(HPMods), [HPMods]
  [OnDesign] -> Scalar_To_Workspace/Enable
  Relational Operator1/1 -> [OnDesign]
  ScalarOutputEnable3/1 -> Relational Operator1/1
  ScalarOutputEnable2/1 -> Relational Operator1/2
  scalarMod/2(C_Eff) -> Bus Creator/11  "s_T_Eff"
  scalarMod/1(C_Wc) -> Bus Creator/9  "s_T_Wc"
  Constant1/1 -> Bus Creator/10  "s_T_PR"
  Constant/1 -> Bus Creator/8  "s_T_Nc"
  [Nmech] -> Bus Creator1/14  "Nmech"
  Block Name from Mask/1 -> Bus Creator1/15  "BlkNm"
  Demux/12 -> Bus Creator1/5  "Wcin"
  PRIn/1 -> Bus Creator/7  "Turbine Pressure Ratio; PRIn[frac]"
  Demux1/2 -> Bus Creator/2  "Turbine Enthalpy; htIn [BTU/lbm]"
  Demux1/3 -> Bus Creator/3  "Turbine Total Temperature; TtIn[degR]"
  Turbine/1 -> Demux/1
  Demux/1 -> Bus Creator2/1  "W"
  Demux/5 -> Bus Creator2/5  "FAR"
  Demux/3 -> Bus Creator2/3  "Tt"
  Demux/4 -> Bus Creator2/4  "Pt"
  Bus Creator/1 -> Turbine/1
  Demux/2 -> Bus Creator2/2  "ht"
  Demux/6 -> TrqOut/1  "Trq"
  Nmech/1 -> Bus Creator/6, [Nmech]  "Turbine Mechanical Shaft Speed; Nmech[rpm]"
  Demux1/4 -> Bus Creator/4  "Turbine Total Pressure; PtIn[psia]"
  Bus Creator2/1 -> GasPthCharOut/1
  GasPthCharIn/1 -> Demux1/1  "Turbine Combusted Fuel to Air Ratio"
  Demux1/1 -> Bus Creator/1  "Turbine Theoretical Gas Flow Input; WIn[pps]"
  Demux/7 -> NErr/1  "NErr"
  CoolingFlwCharIn/1 -> Width/1, Turbine/2  "Cooling Flow Characteristics (W,FAR,Tt,Pt)"
  Demux1/5 -> Bus Creator/5  "Turbine Combusted Fuel to Air Ratio; FARcIn[frac]"
  Bus Creator1/1 -> T_Data/1
  Demux/8 -> Scalar_To_Workspace/1(C_Nc), Bus Creator1/1  "s_T_Nc"
  Demux/9 -> Scalar_To_Workspace/2(C_Wc), Bus Creator1/2  "s_T_Wc"
  Demux/10 -> Scalar_To_Workspace/3(C_PR), Bus Creator1/3  "s_T_PR"
  Demux/11 -> Scalar_To_Workspace/4(C_Eff), Bus Creator1/4  "s_T_Eff"
  Width/1 -> Bus Creator/12  "cfWidth"
  Demux/20 -> Bus Creator1/13  "Test"
  Demux/13 -> Bus Creator1/6  "Wcs1in"
  Demux/14 -> Bus Creator1/7  "Nc"
  Demux/15 -> Bus Creator1/8  "NcMap"
  Demux/16 -> Bus Creator1/9  "WcMap"
  Demux/17 -> Bus Creator1/10  "PRMap"
  Demux/18 -> Bus Creator1/11  "EffMap"
  Demux/19 -> Bus Creator1/12  "Pwrout"

== system O_CloseLoop_Dynmodel/While Iterator Plant/Plant model/Core/S36 Static Calc ==
  S36t : Inport
  Bus Selector2 : BusSelector  OutputSignals=W,ht,Tt,Pt,FAR
  Display : Display
  Display1 : Display
  Mux4 : Mux  Inputs=5
  StaticCalc : Lib_Turbo_StaticCalc_TMATS/StaticCalc  ST_M=off  Ath_M=54  MN_M=1.1  X_FARVec_M=[0; 0.0050; 0.0100; 0.0150; 0.0200; 0.0250; 0.0300]  Y_TtVec_M=[300 10000]  T_RtArray_M="[0.0686;    0.0686;    0.0686;    0.0686;    0.0686;    0.0686;    0.0686]"  T_gammaArray_M=[ 1.4 1.4 1.4 1.4 1.4 1.4 1.4; 1.4 1.4 1.4 1.4 1.4 1.4 1.4]
  S36stc : Outport
  wires:
  Bus Selector2/4 -> Mux4/4  "<Pt>"
  Bus Selector2/2 -> Mux4/2  "<ht>"
  Bus Selector2/5 -> Mux4/5  "<FAR>"
  Bus Selector2/1 -> Mux4/1  "<W>"
  Bus Selector2/3 -> Mux4/3  "<Tt>"
  StaticCalc/1 -> Display/1, S36stc/1
  S36t/1 -> Bus Selector2/1
  Mux4/1 -> Display1/1, StaticCalc/1

== system O_CloseLoop_Dynmodel/While Iterator Plant/Plant model/Core/S36bus ==
  S36tot : Inport
  S36stat : Inport  Port=2
  Bus Creator1 : BusCreator  Inputs=7
  Bus Selector : BusSelector  OutputSignals=Ps,Ts
  Bus Selector1 : BusSelector  OutputSignals=W,ht,Tt,Pt,FAR
  S36all : Outport
  wires:
  Bus Selector1/2 -> Bus Creator1/2  "<ht>"
  Bus Selector1/1 -> Bus Creator1/1  "<W>"
  Bus Selector1/5 -> Bus Creator1/5  "<FAR>"
  Bus Selector/2 -> Bus Creator1/7  "<Ts>"
  S36stat/1 -> Bus Selector/1
  S36tot/1 -> Bus Selector1/1
  Bus Selector/1 -> Bus Creator1/6  "<Ps>"
  Bus Creator1/1 -> S36all/1
  Bus Selector1/3 -> Bus Creator1/3  "<Tt>"
  Bus Selector1/4 -> Bus Creator1/4  "<Pt>"

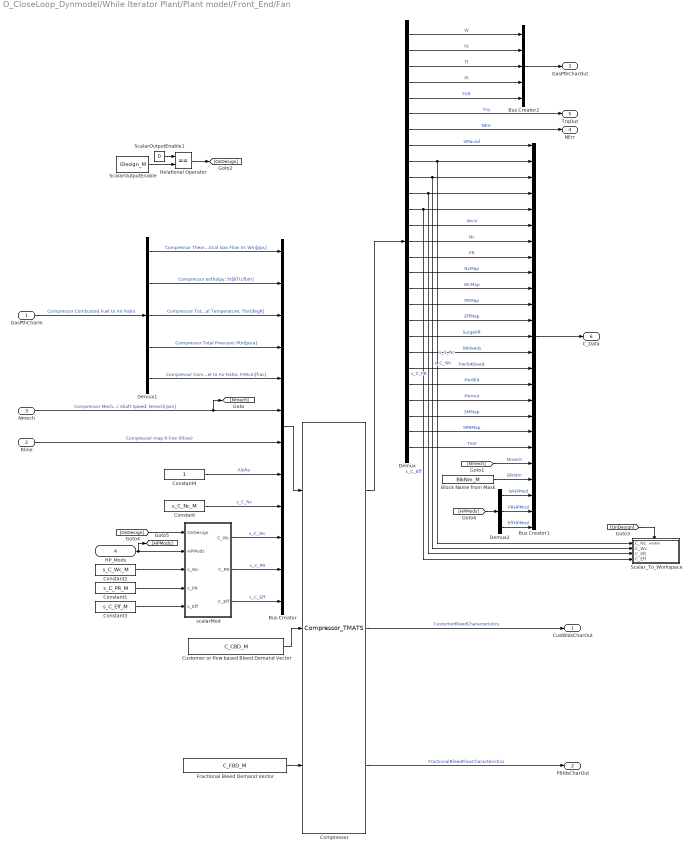
== system O_CloseLoop_Dynmodel/While Iterator Plant/Plant model/Front_End/Fan ==
  GasPthCharIn : Inport
  Rline : Inport  Port=2
  Nmech : Inport  Port=3
  HP_Mods : Inport  Port=4
  Block Name from Mask : Constant  Value=BlkNm_M
  Bus Creator : BusCreator  Inputs=12
  Bus Creator1 : BusCreator  Inputs=25
  Bus Creator2 : BusCreator  Inputs=5
  Compressor : S-Function  FunctionName=Compressor_TMATS  Parameters="Y_C_Map_NcVec_M, X_C_RlineVec_M, Z_C_AlphaVec_M, T_C_Map_WcArray_M, T_C_Map_PRArray_M, T_C_Map_EffArray_M, C_CBFht_M, C_CBFPt_M,  C_BFht_M, C_BFPt_M, X_C_Map_WcSurgeVec_M, T_C_Map_PRSurgeVec_M, iDesign_M, NcDes_M, EffDes_M, PRDes_M, RlineDes_M, CBLDEN_M, FBLDEN_M, gcs, length(C_CBD_M), length(C_FBD_M), size(T_C_Map_WcArray_M,2), size(T_C_Map_PRArray_M,2), size(T_C_Map_EffArray_M,2), size(T_C_Map_WcArray_M,1), size(T_C_Map_PRArray_M,1), size(T_C_Map_EffArray_M,1), size(T_C_Map_WcArray_M,3), size(T_C_Map_PRArray_M,3), size(T_C_Map_EffArray_M,3)"  SFunctionModules='h2tc_TMATS pt2sc_TMATS sp2tc_TMATS t2hc_TMATS interp1Ac_TMATS interp2Ac_TMATS interp3Ac_TMATS functions_TMATS'  SFunctionDeploymentMode=off  EnableBusSupport=off
  Constant : Constant  Value=s_C_Nc_M
  Constant1 : Constant  Value=s_C_PR_M
  Constant2 : Constant  Value=s_C_Wc_M
  Constant3 : Constant  Value=s_C_Eff_M
  Constant4 : Constant
  Customer or flow based Bleed Demand Vector : Constant  Value=C_CBD_M
  Demux : Demux  Outputs=27
  Demux1 : Demux  Outputs=5
  Demux2 : Demux  Outputs=3
  Fractional Bleed Demand Vector : Constant  Value=C_FBD_M
  Relational Operator : RelationalOperator  Operator===  OutDataTypeStr=boolean  RndMeth=Nearest
  ScalarOutputEnable : Constant  Value=iDesign_M
  ScalarOutputEnable1 : Constant  Value=0
  Scalar_To_Workspace : Subsystem
  scalarMod : Subsystem
  CustBldsCharOut : Outport  PortDimensions=length(C_CBD_M)*5
  FBldsCharOut : Outport  Port=2  PortDimensions=length(C_FBD_M)*5
  GasPthCharOut : Outport  Port=3
  NErr : Outport  Port=4
  TrqOut : Outport  Port=5
  C_Data : Outport  Port=6
  wires:
  [HPMods] -> Demux2/1
  Demux2/1 -> Bus Creator1/23  "WHPMod"
  Demux2/3 -> Bus Creator1/25  "EffHPMod"
  Demux2/2 -> Bus Creator1/24  "PRHPMod"
  [OnDesign] -> scalarMod/1(OnDesign)
  HP_Mods/1 -> scalarMod/2(HPMods), [HPMods]
  scalarMod/3(C_Eff) -> Bus Creator/12  "s_C_Eff"
  scalarMod/2(C_PR) -> Bus Creator/11  "s_C_PR"
  scalarMod/1(C_Wc) -> Bus Creator/10  "s_C_Wc"
  Constant3/1 -> scalarMod/5(s_Eff)
  Constant1/1 -> scalarMod/4(s_PR)
  Constant2/1 -> scalarMod/3(s_Wc)
  [OnDesign] -> Scalar_To_Workspace/Enable
  Constant4/1 -> Bus Creator/8  "Alpha"
  Constant/1 -> Bus Creator/9  "s_C_Nc"
  Block Name from Mask/1 -> Bus Creator1/22  "BlkNm"
  [Nmech] -> Bus Creator1/21  "Nmech"
  Demux/27 -> Bus Creator1/20  "Test"
  Demux/26 -> Bus Creator1/19  "SPRMap"
  Demux/25 -> Bus Creator1/18  "SMMap"
  Demux/18 -> Bus Creator1/11  "PRMap"
  Demux/15 -> Bus Creator1/8  "PR"
  Demux/17 -> Bus Creator1/10  "WcMap"
  Demux/19 -> Bus Creator1/12  "EffMap"
  Demux/24 -> Bus Creator1/17  "Pwrout"
  Demux/16 -> Bus Creator1/9  "NcMap"
  Demux/20 -> Bus Creator1/13  "SurgePR"
  Demux/21 -> Bus Creator1/14  "Wbleeds"
  Demux/22 -> Bus Creator1/15  "Pwrb4bleed"
  Demux/23 -> Bus Creator1/16  "PwrBld"
  Demux/14 -> Bus Creator1/7  "Nc"
  Relational Operator/1 -> [OnDesign]
  ScalarOutputEnable1/1 -> Relational Operator/1
  ScalarOutputEnable/1 -> Relational Operator/2
  Demux/12 -> Bus Creator1/5, Scalar_To_Workspace/4(C_Eff)  "s_C_Eff"
  Demux/11 -> Bus Creator1/4, Scalar_To_Workspace/3(C_PR)  "s_C_PR"
  Demux/10 -> Bus Creator1/3, Scalar_To_Workspace/2(C_Wc)  "s_C_Wc"
  Demux/9 -> Bus Creator1/2, Scalar_To_Workspace/1(C_Nc)  "s_C_Nc"
  Bus Creator1/1 -> C_Data/1
  Demux/8 -> Bus Creator1/1  "SMavail"
  Demux1/2 -> Bus Creator/2  "Compressor enthalpy; ht[BTU/lbm]"
  Compressor/3 -> FBldsCharOut/1  "FractionalBleedFlowCharacteristics"
  Compressor/2 -> CustBldsCharOut/1  "CustomerBleedCharacteristics"
  Fractional Bleed Demand Vector/1 -> Compressor/3
  Customer or flow based Bleed Demand Vector/1 -> Compressor/2
  Demux/7 -> NErr/1  "NErr"
  Demux1/1 -> Bus Creator/1  "Compressor Theoretical Gas Flow In; WIn[pps]"
  GasPthCharIn/1 -> Demux1/1  "Compressor Combusted Fuel to Air Ratio"
  Bus Creator2/1 -> GasPthCharOut/1
  Demux/2 -> Bus Creator2/2  "ht"
  Demux/13 -> Bus Creator1/6  "Wcin"
  Rline/1 -> Bus Creator/7  "Compressor map R-line (Rline)"
  Demux1/5 -> Bus Creator/5  "Compressor Combusted Fuel to Air Ratio; FARcIn[frac]"
  Demux1/3 -> Bus Creator/3  "Compressor Total Temperature; TtIn[degR]"
  Compressor/1 -> Demux/1
  Demux/1 -> Bus Creator2/1  "W"
  Demux/5 -> Bus Creator2/5  "FAR"
  Demux/3 -> Bus Creator2/3  "Tt"
  Demux/4 -> Bus Creator2/4  "Pt"
  Bus Creator/1 -> Compressor/1
  Demux/6 -> TrqOut/1  "Trq"
  Nmech/1 -> Bus Creator/6, [Nmech]  "Compressor Mechanical Shaft Speed; Nmech[rpm]"
  Demux1/4 -> Bus Creator/4  "Compressor Total Pressure; PtIn[psia]"

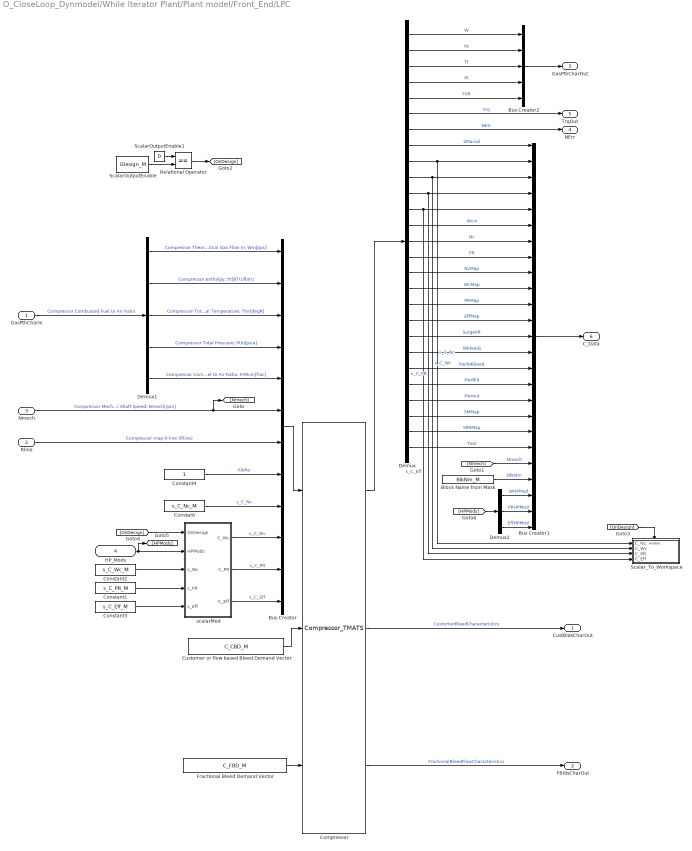
== system O_CloseLoop_Dynmodel/While Iterator Plant/Plant model/Front_End/LPC ==
  GasPthCharIn : Inport
  Rline : Inport  Port=2
  Nmech : Inport  Port=3
  HP_Mods : Inport  Port=4
  Block Name from Mask : Constant  Value=BlkNm_M
  Bus Creator : BusCreator  Inputs=12
  Bus Creator1 : BusCreator  Inputs=25
  Bus Creator2 : BusCreator  Inputs=5
  Compressor : S-Function  FunctionName=Compressor_TMATS  Parameters="Y_C_Map_NcVec_M, X_C_RlineVec_M, Z_C_AlphaVec_M, T_C_Map_WcArray_M, T_C_Map_PRArray_M, T_C_Map_EffArray_M, C_CBFht_M, C_CBFPt_M,  C_BFht_M, C_BFPt_M, X_C_Map_WcSurgeVec_M, T_C_Map_PRSurgeVec_M, iDesign_M, NcDes_M, EffDes_M, PRDes_M, RlineDes_M, CBLDEN_M, FBLDEN_M, gcs, length(C_CBD_M), length(C_FBD_M), size(T_C_Map_WcArray_M,2), size(T_C_Map_PRArray_M,2), size(T_C_Map_EffArray_M,2), size(T_C_Map_WcArray_M,1), size(T_C_Map_PRArray_M,1), size(T_C_Map_EffArray_M,1), size(T_C_Map_WcArray_M,3), size(T_C_Map_PRArray_M,3), size(T_C_Map_EffArray_M,3)"  SFunctionModules='h2tc_TMATS pt2sc_TMATS sp2tc_TMATS t2hc_TMATS interp1Ac_TMATS interp2Ac_TMATS interp3Ac_TMATS functions_TMATS'  SFunctionDeploymentMode=off  EnableBusSupport=off
  Constant : Constant  Value=s_C_Nc_M
  Constant1 : Constant  Value=s_C_PR_M
  Constant2 : Constant  Value=s_C_Wc_M
  Constant3 : Constant  Value=s_C_Eff_M
  Constant4 : Constant
  Customer or flow based Bleed Demand Vector : Constant  Value=C_CBD_M
  Demux : Demux  Outputs=27
  Demux1 : Demux  Outputs=5
  Demux2 : Demux  Outputs=3
  Fractional Bleed Demand Vector : Constant  Value=C_FBD_M
  Relational Operator : RelationalOperator  Operator===  OutDataTypeStr=boolean  RndMeth=Nearest
  ScalarOutputEnable : Constant  Value=iDesign_M
  ScalarOutputEnable1 : Constant  Value=0
  Scalar_To_Workspace : Subsystem
  scalarMod : Subsystem
  CustBldsCharOut : Outport  PortDimensions=length(C_CBD_M)*5
  FBldsCharOut : Outport  Port=2  PortDimensions=length(C_FBD_M)*5
  GasPthCharOut : Outport  Port=3
  NErr : Outport  Port=4
  TrqOut : Outport  Port=5
  C_Data : Outport  Port=6
  wires:
  [HPMods] -> Demux2/1
  Demux2/1 -> Bus Creator1/23  "WHPMod"
  Demux2/3 -> Bus Creator1/25  "EffHPMod"
  Demux2/2 -> Bus Creator1/24  "PRHPMod"
  [OnDesign] -> scalarMod/1(OnDesign)
  HP_Mods/1 -> scalarMod/2(HPMods), [HPMods]
  scalarMod/3(C_Eff) -> Bus Creator/12  "s_C_Eff"
  scalarMod/2(C_PR) -> Bus Creator/11  "s_C_PR"
  scalarMod/1(C_Wc) -> Bus Creator/10  "s_C_Wc"
  Constant3/1 -> scalarMod/5(s_Eff)
  Constant1/1 -> scalarMod/4(s_PR)
  Constant2/1 -> scalarMod/3(s_Wc)
  [OnDesign] -> Scalar_To_Workspace/Enable
  Constant4/1 -> Bus Creator/8  "Alpha"
  Constant/1 -> Bus Creator/9  "s_C_Nc"
  Block Name from Mask/1 -> Bus Creator1/22  "BlkNm"
  [Nmech] -> Bus Creator1/21  "Nmech"
  Demux/27 -> Bus Creator1/20  "Test"
  Demux/26 -> Bus Creator1/19  "SPRMap"
  Demux/25 -> Bus Creator1/18  "SMMap"
  Demux/18 -> Bus Creator1/11  "PRMap"
  Demux/15 -> Bus Creator1/8  "PR"
  Demux/17 -> Bus Creator1/10  "WcMap"
  Demux/19 -> Bus Creator1/12  "EffMap"
  Demux/24 -> Bus Creator1/17  "Pwrout"
  Demux/16 -> Bus Creator1/9  "NcMap"
  Demux/20 -> Bus Creator1/13  "SurgePR"
  Demux/21 -> Bus Creator1/14  "Wbleeds"
  Demux/22 -> Bus Creator1/15  "Pwrb4bleed"
  Demux/23 -> Bus Creator1/16  "PwrBld"
  Demux/14 -> Bus Creator1/7  "Nc"
  Relational Operator/1 -> [OnDesign]
  ScalarOutputEnable1/1 -> Relational Operator/1
  ScalarOutputEnable/1 -> Relational Operator/2
  Demux/12 -> Bus Creator1/5, Scalar_To_Workspace/4(C_Eff)  "s_C_Eff"
  Demux/11 -> Bus Creator1/4, Scalar_To_Workspace/3(C_PR)  "s_C_PR"
  Demux/10 -> Bus Creator1/3, Scalar_To_Workspace/2(C_Wc)  "s_C_Wc"
  Demux/9 -> Bus Creator1/2, Scalar_To_Workspace/1(C_Nc)  "s_C_Nc"
  Bus Creator1/1 -> C_Data/1
  Demux/8 -> Bus Creator1/1  "SMavail"
  Demux1/2 -> Bus Creator/2  "Compressor enthalpy; ht[BTU/lbm]"
  Compressor/3 -> FBldsCharOut/1  "FractionalBleedFlowCharacteristics"
  Compressor/2 -> CustBldsCharOut/1  "CustomerBleedCharacteristics"
  Fractional Bleed Demand Vector/1 -> Compressor/3
  Customer or flow based Bleed Demand Vector/1 -> Compressor/2
  Demux/7 -> NErr/1  "NErr"
  Demux1/1 -> Bus Creator/1  "Compressor Theoretical Gas Flow In; WIn[pps]"
  GasPthCharIn/1 -> Demux1/1  "Compressor Combusted Fuel to Air Ratio"
  Bus Creator2/1 -> GasPthCharOut/1
  Demux/2 -> Bus Creator2/2  "ht"
  Demux/13 -> Bus Creator1/6  "Wcin"
  Rline/1 -> Bus Creator/7  "Compressor map R-line (Rline)"
  Demux1/5 -> Bus Creator/5  "Compressor Combusted Fuel to Air Ratio; FARcIn[frac]"
  Demux1/3 -> Bus Creator/3  "Compressor Total Temperature; TtIn[degR]"
  Compressor/1 -> Demux/1
  Demux/1 -> Bus Creator2/1  "W"
  Demux/5 -> Bus Creator2/5  "FAR"
  Demux/3 -> Bus Creator2/3  "Tt"
  Demux/4 -> Bus Creator2/4  "Pt"
  Bus Creator/1 -> Compressor/1
  Demux/6 -> TrqOut/1  "Trq"
  Nmech/1 -> Bus Creator/6, [Nmech]  "Compressor Mechanical Shaft Speed; Nmech[rpm]"
  Demux1/4 -> Bus Creator/4  "Compressor Total Pressure; PtIn[psia]"

== system O_CloseLoop_Dynmodel/While Iterator Plant/Plant model/Back_Eng/LPT/Scalar_To_Workspace ==
  C_Nc : Inport
  C_Wc : Inport  Port=2
  C_PR : Inport  Port=3
  C_Eff : Inport  Port=4
  Enable : EnablePort
  DataOutput : Lib_Solve_DataOut_TMATS/DataOutput  FVar_M=double(FVar_M)
  Mux : Mux
  wires:
  C_Wc/1 -> Mux/2
  C_Nc/1 -> Mux/1
  C_PR/1 -> Mux/3
  C_Eff/1 -> Mux/4
  Mux/1 -> DataOutput/1

== system O_CloseLoop_Dynmodel/While Iterator Plant/Plant model/Back_Eng/LPT/scalarMod ==
  OnDesign : Inport
  HPMods : Inport  Port=2
  s_Wc : Inport  Port=3
  s_Eff : Inport  Port=4
  Constant : Constant
  Constant2 : Constant
  Data Type Conversion : DataTypeConversion
  Demux : Demux  Outputs=2
  Logical Operator : Logic  Operator=NOT  AllPortsSameDT=off  OutDataTypeStr=boolean
  Product{,3..5} (4 alike) : Product
  Sum : Sum  Inputs=++|
  Sum2 : Sum  Inputs=++|
  C_Wc : Outport
  C_Eff : Outport  Port=2
  wires:
  Product4/1 -> C_Eff/1  "s_C_Eff"
  Product/1 -> C_Wc/1  "s_C_Wc"
  s_Wc/1 -> Product/2
  OnDesign/1 -> Logical Operator/1
  Data Type Conversion/1 -> [OffDesign]
  Logical Operator/1 -> Data Type Conversion/1
  Sum/1 -> Product/1
  [WcMod] -> Product3/1
  Constant/1 -> Sum/1
  Product3/1 -> Sum/2
  [OffDesign] -> Product3/2
  s_Eff/1 -> Product4/2
  Sum2/1 -> Product4/1
  [EffMod] -> Product5/1
  Constant2/1 -> Sum2/1
  Product5/1 -> Sum2/2
  [OffDesign] -> Product5/2
  HPMods/1 -> Demux/1
  Demux/1 -> [WcMod]
  Demux/2 -> [EffMod]

== system O_CloseLoop_Dynmodel/While Iterator Plant/Plant model/Core/HPC/Scalar_To_Workspace ==
  C_Nc : Inport
  C_Wc : Inport  Port=2
  C_PR : Inport  Port=3
  C_Eff : Inport  Port=4
  Enable : EnablePort
  DataOutput : Lib_Solve_DataOut_TMATS/DataOutput  FVar_M=double(FVar_M)
  Mux : Mux
  wires:
  Mux/1 -> DataOutput/1
  C_Eff/1 -> Mux/4
  C_PR/1 -> Mux/3
  C_Wc/1 -> Mux/2
  C_Nc/1 -> Mux/1

== system O_CloseLoop_Dynmodel/While Iterator Plant/Plant model/Core/HPC/scalarMod ==
  OnDesign : Inport
  HPMods : Inport  Port=2
  s_Wc : Inport  Port=3
  s_PR : Inport  Port=4
  s_Eff : Inport  Port=5
  Constant : Constant
  Constant1 : Constant
  Constant2 : Constant
  Data Type Conversion : DataTypeConversion
  Demux : Demux  Outputs=3
  Logical Operator : Logic  Operator=NOT  AllPortsSameDT=off  OutDataTypeStr=boolean
  Product{,1..5} (6 alike) : Product
  Sum : Sum  Inputs=++|
  Sum1 : Sum  Inputs=++|
  Sum2 : Sum  Inputs=++|
  C_Wc : Outport
  C_PR : Outport  Port=2
  C_Eff : Outport  Port=3
  wires:
  Demux/3 -> [EffMod]
  Demux/2 -> [PRMod]
  Demux/1 -> [WcMod]
  HPMods/1 -> Demux/1
  [OffDesign] -> Product5/2
  Product5/1 -> Sum2/2
  Constant2/1 -> Sum2/1
  [EffMod] -> Product5/1
  Sum2/1 -> Product4/1
  s_Eff/1 -> Product4/2
  [OffDesign] -> Product2/2
  Product2/1 -> Sum1/2
  Constant1/1 -> Sum1/1
  [PRMod] -> Product2/1
  Sum1/1 -> Product1/1
  s_PR/1 -> Product1/2
  [OffDesign] -> Product3/2
  Product3/1 -> Sum/2
  Constant/1 -> Sum/1
  [WcMod] -> Product3/1
  Sum/1 -> Product/1
  Logical Operator/1 -> Data Type Conversion/1
  Data Type Conversion/1 -> [OffDesign]
  OnDesign/1 -> Logical Operator/1
  s_Wc/1 -> Product/2
  Product/1 -> C_Wc/1  "s_C_Wc"
  Product4/1 -> C_Eff/1  "s_C_Eff"
  Product1/1 -> C_PR/1  "s_C_PR"

== system O_CloseLoop_Dynmodel/While Iterator Plant/Plant model/Core/HPT/Scalar_To_Workspace ==
  C_Nc : Inport
  C_Wc : Inport  Port=2
  C_PR : Inport  Port=3
  C_Eff : Inport  Port=4
  Enable : EnablePort
  DataOutput : Lib_Solve_DataOut_TMATS/DataOutput  FVar_M=double(FVar_M)
  Mux : Mux
  wires:
  C_Wc/1 -> Mux/2
  C_Nc/1 -> Mux/1
  C_PR/1 -> Mux/3
  C_Eff/1 -> Mux/4
  Mux/1 -> DataOutput/1

== system O_CloseLoop_Dynmodel/While Iterator Plant/Plant model/Core/HPT/scalarMod ==
  OnDesign : Inport
  HPMods : Inport  Port=2
  s_Wc : Inport  Port=3
  s_Eff : Inport  Port=4
  Constant : Constant
  Constant2 : Constant
  Data Type Conversion : DataTypeConversion
  Demux : Demux  Outputs=2
  Logical Operator : Logic  Operator=NOT  AllPortsSameDT=off  OutDataTypeStr=boolean
  Product{,3..5} (4 alike) : Product
  Sum : Sum  Inputs=++|
  Sum2 : Sum  Inputs=++|
  C_Wc : Outport
  C_Eff : Outport  Port=2
  wires:
  Product4/1 -> C_Eff/1  "s_C_Eff"
  Product/1 -> C_Wc/1  "s_C_Wc"
  s_Wc/1 -> Product/2
  OnDesign/1 -> Logical Operator/1
  Data Type Conversion/1 -> [OffDesign]
  Logical Operator/1 -> Data Type Conversion/1
  Sum/1 -> Product/1
  [WcMod] -> Product3/1
  Constant/1 -> Sum/1
  Product3/1 -> Sum/2
  [OffDesign] -> Product3/2
  s_Eff/1 -> Product4/2
  Sum2/1 -> Product4/1
  [EffMod] -> Product5/1
  Constant2/1 -> Sum2/1
  Product5/1 -> Sum2/2
  [OffDesign] -> Product5/2
  HPMods/1 -> Demux/1
  Demux/1 -> [WcMod]
  Demux/2 -> [EffMod]

== system O_CloseLoop_Dynmodel/While Iterator Plant/Plant model/Front_End/Fan/Scalar_To_Workspace ==
  C_Nc : Inport
  C_Wc : Inport  Port=2
  C_PR : Inport  Port=3
  C_Eff : Inport  Port=4
  Enable : EnablePort
  DataOutput : Lib_Solve_DataOut_TMATS/DataOutput  FVar_M=double(FVar_M)
  Mux : Mux
  wires:
  Mux/1 -> DataOutput/1
  C_Eff/1 -> Mux/4
  C_PR/1 -> Mux/3
  C_Wc/1 -> Mux/2
  C_Nc/1 -> Mux/1

== system O_CloseLoop_Dynmodel/While Iterator Plant/Plant model/Front_End/Fan/scalarMod ==
  OnDesign : Inport
  HPMods : Inport  Port=2
  s_Wc : Inport  Port=3
  s_PR : Inport  Port=4
  s_Eff : Inport  Port=5
  Constant : Constant
  Constant1 : Constant
  Constant2 : Constant
  Data Type Conversion : DataTypeConversion
  Demux : Demux  Outputs=3
  Logical Operator : Logic  Operator=NOT  AllPortsSameDT=off  OutDataTypeStr=boolean
  Product{,1..5} (6 alike) : Product
  Sum : Sum  Inputs=++|
  Sum1 : Sum  Inputs=++|
  Sum2 : Sum  Inputs=++|
  C_Wc : Outport
  C_PR : Outport  Port=2
  C_Eff : Outport  Port=3
  wires:
  Demux/3 -> [EffMod]
  Demux/2 -> [PRMod]
  Demux/1 -> [WcMod]
  HPMods/1 -> Demux/1
  [OffDesign] -> Product5/2
  Product5/1 -> Sum2/2
  Constant2/1 -> Sum2/1
  [EffMod] -> Product5/1
  Sum2/1 -> Product4/1
  s_Eff/1 -> Product4/2
  [OffDesign] -> Product2/2
  Product2/1 -> Sum1/2
  Constant1/1 -> Sum1/1
  [PRMod] -> Product2/1
  Sum1/1 -> Product1/1
  s_PR/1 -> Product1/2
  [OffDesign] -> Product3/2
  Product3/1 -> Sum/2
  Constant/1 -> Sum/1
  [WcMod] -> Product3/1
  Sum/1 -> Product/1
  Logical Operator/1 -> Data Type Conversion/1
  Data Type Conversion/1 -> [OffDesign]
  OnDesign/1 -> Logical Operator/1
  s_Wc/1 -> Product/2
  Product/1 -> C_Wc/1  "s_C_Wc"
  Product4/1 -> C_Eff/1  "s_C_Eff"
  Product1/1 -> C_PR/1  "s_C_PR"

== system O_CloseLoop_Dynmodel/While Iterator Plant/Plant model/Front_End/LPC/Scalar_To_Workspace ==
  C_Nc : Inport
  C_Wc : Inport  Port=2
  C_PR : Inport  Port=3
  C_Eff : Inport  Port=4
  Enable : EnablePort
  DataOutput : Lib_Solve_DataOut_TMATS/DataOutput  FVar_M=double(FVar_M)
  Mux : Mux
  wires:
  Mux/1 -> DataOutput/1
  C_Eff/1 -> Mux/4
  C_PR/1 -> Mux/3
  C_Wc/1 -> Mux/2
  C_Nc/1 -> Mux/1

== system O_CloseLoop_Dynmodel/While Iterator Plant/Plant model/Front_End/LPC/scalarMod ==
  OnDesign : Inport
  HPMods : Inport  Port=2
  s_Wc : Inport  Port=3
  s_PR : Inport  Port=4
  s_Eff : Inport  Port=5
  Constant : Constant
  Constant1 : Constant
  Constant2 : Constant
  Data Type Conversion : DataTypeConversion
  Demux : Demux  Outputs=3
  Logical Operator : Logic  Operator=NOT  AllPortsSameDT=off  OutDataTypeStr=boolean
  Product{,1..5} (6 alike) : Product
  Sum : Sum  Inputs=++|
  Sum1 : Sum  Inputs=++|
  Sum2 : Sum  Inputs=++|
  C_Wc : Outport
  C_PR : Outport  Port=2
  C_Eff : Outport  Port=3
  wires:
  Demux/3 -> [EffMod]
  Demux/2 -> [PRMod]
  Demux/1 -> [WcMod]
  HPMods/1 -> Demux/1
  [OffDesign] -> Product5/2
  Product5/1 -> Sum2/2
  Constant2/1 -> Sum2/1
  [EffMod] -> Product5/1
  Sum2/1 -> Product4/1
  s_Eff/1 -> Product4/2
  [OffDesign] -> Product2/2
  Product2/1 -> Sum1/2
  Constant1/1 -> Sum1/1
  [PRMod] -> Product2/1
  Sum1/1 -> Product1/1
  s_PR/1 -> Product1/2
  [OffDesign] -> Product3/2
  Product3/1 -> Sum/2
  Constant/1 -> Sum/1
  [WcMod] -> Product3/1
  Sum/1 -> Product/1
  Logical Operator/1 -> Data Type Conversion/1
  Data Type Conversion/1 -> [OffDesign]
  OnDesign/1 -> Logical Operator/1
  s_Wc/1 -> Product/2
  Product/1 -> C_Wc/1  "s_C_Wc"
  Product4/1 -> C_Eff/1  "s_C_Eff"
  Product1/1 -> C_PR/1  "s_C_PR"
